simulink model "pmdc_and_series_motor_tr"  (R2016a)
settings: Solver=ode45  StartTime=0.0  StopTime=1  RelTol=1e-3
values from neighbouring files (symbols this model uses):
  Dm_PMDC = 6.01e-6    (= 6.01e-06)    [init_params_PMDC_Series.m]
  Dm_SS = 6.01e-6    (= 6.01e-06)    [init_params_PMDC_Series.m]
  J_PMDC = 1.06e-6    (= 1.06e-06)    [init_params_PMDC_Series.m]
  J_SS = 1.06e-6    (= 1.06e-06)    [init_params_PMDC_Series.m]
  Kv_PMDC = 0.0141    [init_params_PMDC_Series.m]
  Laf_SS = 21.6/1000    (= 0.0216)    [init_params_PMDC_Series.m]
  Ra_PMDC = 7    [init_params_PMDC_Series.m]
  Ra_SS = 7    [init_params_PMDC_Series.m]
  Rf_SS = 0.12    [init_params_PMDC_Series.m]
  Ta_PMDC = La_PMDC/Ra_PMDC    (= 0.00171428571429)    [init_params_PMDC_Series.m]
  Tfa_SS = La_SS/Ra_SS    (= 0.00171428571429)    [init_params_PMDC_Series.m]
  Tm_PMDC = 3.53e-3    (= 0.00353)    [init_params_PMDC_Series.m]
  Tm_SS = 3.53e-3    (= 0.00353)    [init_params_PMDC_Series.m]
  Va_PMDC = 6    [init_params_PMDC_Series.m]
  Va_SS = 6    [init_params_PMDC_Series.m]
settings Model: Creator=Atif Ali  LastModifiedBy=asali
settings DataIOCC: SaveFormat=Array
settings DebuggingCC: UnderspecifiedInitializationDetection=Classic  MergeDetectMultiDrivingBlocksExec=none
settings HardwareCC: ProdBitPerPointer=32  ProdLargestAtomicFloat=None  ProdIntDivRoundTo=Undefined  ProdEndianess=Unspecified  ProdWordSize=32  ProdHWDeviceType=32-bit Generic
settings ModelReferenceCC: PropagateSignalLabelsOutOfModel=off
settings ConfigComp: CovModelRefEnable=Off

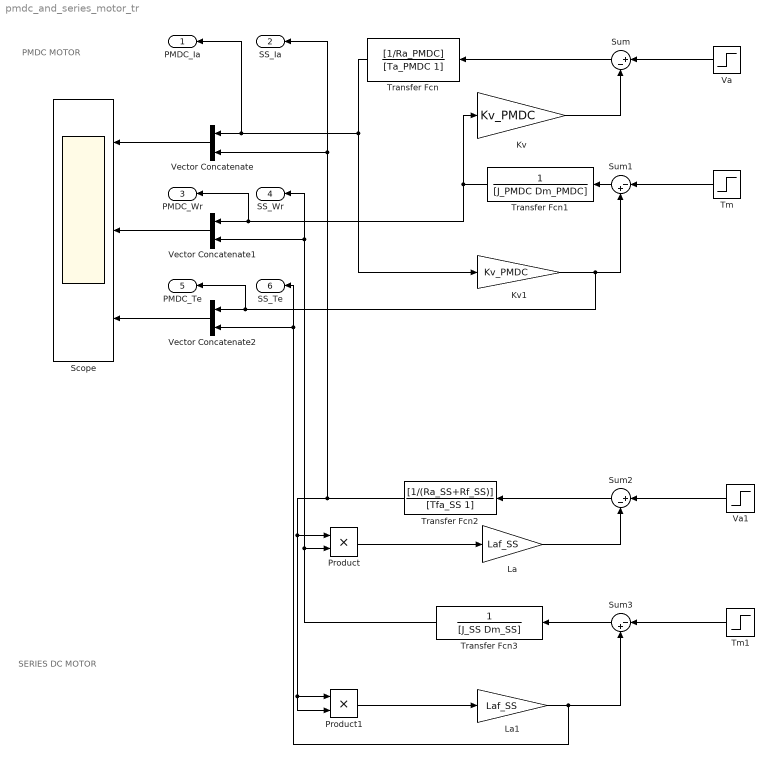
== system pmdc_and_series_motor_tr ==
  note: SERIES DC MOTOR
  note: PMDC MOTOR
  Kv : Gain  Gain=Kv_PMDC
  Kv1 : Gain  Gain=Kv_PMDC
  La : Gain  Gain=Laf_SS
  La1 : Gain  Gain=Laf_SS
  Product : Product
  Product1 : Product
  Scope : Scope  NumInputPorts=3
  Sum : Sum  Inputs=|+-
  Sum1 : Sum  Inputs=|-+
  Sum2 : Sum  Inputs=|+-
  Sum3 : Sum  Inputs=|-+
  Tm : Step  Time=0.5  After=Tm_PMDC  SampleTime=0
  Tm1 : Step  Time=0.5  After=Tm_SS  SampleTime=0
  Transfer Fcn : TransferFcn  Numerator=[1/Ra_PMDC]  Denominator=[Ta_PMDC 1]
  Transfer Fcn1 : TransferFcn  Denominator=[J_PMDC Dm_PMDC]
  Transfer Fcn2 : TransferFcn  Numerator=[1/(Ra_SS+Rf_SS)]  Denominator=[Tfa_SS 1]
  Transfer Fcn3 : TransferFcn  Denominator=[J_SS Dm_SS]
  Va : Step  Time=0.05  After=Va_PMDC  SampleTime=0
  Va1 : Step  Time=0.05  After=Va_SS  SampleTime=0
  Vector Concatenate : Concatenate
  Vector Concatenate1 : Concatenate
  Vector Concatenate2 : Concatenate
  PMDC_Ia : Outport
  SS_Ia : Outport  Port=2
  PMDC_Wr : Outport  Port=3
  SS_Wr : Outport  Port=4
  PMDC_Te : Outport  Port=5
  SS_Te : Outport  Port=6
  wires:
  Sum/1 -> Transfer Fcn/1
  Transfer Fcn/1 -> PMDC_Ia/1, Vector Concatenate/1, Kv1/1
  Kv1/1 -> Sum1/2, PMDC_Te/1, Vector Concatenate2/1
  Kv/1 -> Sum/2
  Sum1/1 -> Transfer Fcn1/1
  Transfer Fcn1/1 -> Kv/1, PMDC_Wr/1, Vector Concatenate1/1
  Va/1 -> Sum/1
  Tm/1 -> Sum1/1
  Sum2/1 -> Transfer Fcn2/1
  La1/1 -> SS_Te/1, Vector Concatenate2/2, Sum3/2
  La/1 -> Sum2/2
  Sum3/1 -> Transfer Fcn3/1
  Product/1 -> La/1
  Transfer Fcn2/1 -> SS_Ia/1, Vector Concatenate/2, Product1/2, Product1/1, Product/1
  Transfer Fcn3/1 -> SS_Wr/1, Vector Concatenate1/2, Product/2
  Product1/1 -> La1/1
  Vector Concatenate/1 -> Scope/1
  Vector Concatenate1/1 -> Scope/2
  Vector Concatenate2/1 -> Scope/3
  Tm1/1 -> Sum3/1
  Va1/1 -> Sum2/1
